simulink model "Exercise21"  (R2016a)
settings: Solver=VariableStepAuto  StartTime=0.0  StopTime=10.0  RelTol=1e-3
values from neighbouring files (symbols this model uses):
  A = 1    [Exercise2.m]
  f0 = 100*1e3    (= 100000)    [Exercise2.m]
  Ts = 1/Fs    (= 1e-06)    [Exercise2.m]
undefined symbols (not defined in the file or in its folder): den, num
settings Model: Creator=sergi  LastModifiedBy=sergi

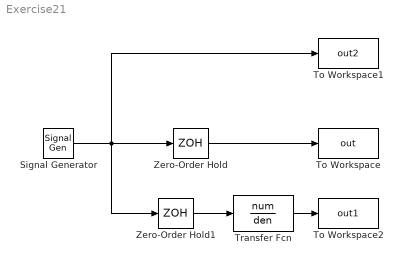
== system Exercise21 ==
  Signal Generator : SignalGenerator  Amplitude=A  Frequency=f0
  To Workspace : ToWorkspace  VariableName=out  SampleTime=Ts/10
      settings: Save2DSignal=2-D array (concatenate along first dimension)
  To Workspace1 : ToWorkspace  VariableName=out2  SampleTime=Ts
      settings: Save2DSignal=2-D array (concatenate along first dimension)
  To Workspace2 : ToWorkspace  VariableName=out1  SampleTime=Ts/10
      settings: Save2DSignal=2-D array (concatenate along first dimension)
  Transfer Fcn : TransferFcn  Numerator=num  Denominator=den
  Zero-Order Hold : ZeroOrderHold  SampleTime=Ts
  Zero-Order Hold1 : ZeroOrderHold  SampleTime=Ts
  wires:
  Signal Generator/1 -> To Workspace1/1, Zero-Order Hold1/1, Zero-Order Hold/1
  Zero-Order Hold/1 -> To Workspace/1
  Zero-Order Hold1/1 -> Transfer Fcn/1
  Transfer Fcn/1 -> To Workspace2/1
